simulink model "Rail_CtlLoop"  (R2016b)
settings: configuration reference "CodeGenConfigSet" (kept outside this file)
values from neighbouring files (symbols this model uses):
  FlSys_stDeflate_C = Calibration.Parameter    [init_Rail_CtlLoop.m]    (also in init_Rail_CtlLoop_SIL.m = Simulink.Parameter)
  Rail_dvolMeUnCtlInitI_CUR = Calibration.Parameter    [init_Rail_CtlLoop.m]    (also in init_Rail_CtlLoop_SIL.m = Simulink.Parameter)
  Rail_dvolMeUnCtlInitI_CURX = Calibration.Parameter    [init_Rail_CtlLoop.m]    (also in init_Rail_CtlLoop_SIL.m = Simulink.Parameter)
  Rail_dvolMeUnCtlLoLim_C = Calibration.Parameter    [init_Rail_CtlLoop.m]    (also in init_Rail_CtlLoop_SIL.m = Simulink.Parameter)
  Rail_dvolOff_C = Calibration.Parameter    [init_Rail_CtlLoop.m]    (also in init_Rail_CtlLoop_SIL.m = Simulink.Parameter)
  Rail_dvolPRVCtlOfs_C = Calibration.Parameter    [init_Rail_CtlLoop.m]    (also in init_Rail_CtlLoop_SIL.m = Simulink.Parameter)
  Rail_dvolStrt_MAP = Calibration.Parameter    [init_Rail_CtlLoop.m]    (also in init_Rail_CtlLoop_SIL.m = Simulink.Parameter)
  Rail_dvolStrt_MAPX = Calibration.Parameter    [init_Rail_CtlLoop.m]    (also in init_Rail_CtlLoop_SIL.m = Simulink.Parameter)
  Rail_dvolStrt_MAPY = Calibration.Parameter    [init_Rail_CtlLoop.m]    (also in init_Rail_CtlLoop_SIL.m = Simulink.Parameter)
  Rail_nCloseCtl_C = Calibration.Parameter    [init_Rail_CtlLoop.m]    (also in init_Rail_CtlLoop_SIL.m = Simulink.Parameter)
  Rail_nMeUnFrzI_C = Calibration.Parameter    [init_Rail_CtlLoop.m]    (also in init_Rail_CtlLoop_SIL.m = Simulink.Parameter)
  Rail_nOpnCtl_C = Calibration.Parameter    [init_Rail_CtlLoop.m]    (also in init_Rail_CtlLoop_SIL.m = Simulink.Parameter)
  Rail_nStrtLoPress_C = Calibration.Parameter    [init_Rail_CtlLoop.m]    (also in init_Rail_CtlLoop_SIL.m = Simulink.Parameter)
  Rail_numRevPlaus_C = Calibration.Parameter    [init_Rail_CtlLoop.m]    (also in init_Rail_CtlLoop_SIL.m = Simulink.Parameter)
  Rail_pCloseCtl_C = Calibration.Parameter    [init_Rail_CtlLoop.m]    (also in init_Rail_CtlLoop_SIL.m = Simulink.Parameter)
  Rail_pDiffCloseCtl_C = Calibration.Parameter    [init_Rail_CtlLoop.m]    (also in init_Rail_CtlLoop_SIL.m = Simulink.Parameter)
  Rail_pDvtFltMin_C = Calibration.Parameter    [init_Rail_CtlLoop.m]    (also in init_Rail_CtlLoop_SIL.m = Simulink.Parameter)
  Rail_pMeUnCtlIWinNeg_C = Calibration.Parameter    [init_Rail_CtlLoop.m]    (also in init_Rail_CtlLoop_SIL.m = Simulink.Parameter)
  Rail_pMeUnCtlIWinPos_C = Calibration.Parameter    [init_Rail_CtlLoop.m]    (also in init_Rail_CtlLoop_SIL.m = Simulink.Parameter)
  Rail_pMeUnCtlPWinNeg_C = Calibration.Parameter    [init_Rail_CtlLoop.m]    (also in init_Rail_CtlLoop_SIL.m = Simulink.Parameter)
  Rail_pMeUnCtlPWinPos_C = Calibration.Parameter    [init_Rail_CtlLoop.m]    (also in init_Rail_CtlLoop_SIL.m = Simulink.Parameter)
  Rail_pOpnCtl_C = Calibration.Parameter    [init_Rail_CtlLoop.m]    (also in init_Rail_CtlLoop_SIL.m = Simulink.Parameter)
  Rail_stCtlLoopSel_C = Calibration.Parameter    [init_Rail_CtlLoop.m]    (also in init_Rail_CtlLoop_SIL.m = Simulink.Parameter)
  Rail_swtPress_C = Calibration.Parameter    [init_Rail_CtlLoop.m]    (also in init_Rail_CtlLoop_SIL.m = Simulink.Parameter)
  Rail_tiFrzIDel_C = Calibration.Parameter    [init_Rail_CtlLoop.m]    (also in init_Rail_CtlLoop_SIL.m = Simulink.Parameter)
undefined symbols (not defined in the file or in its folder): Rail_CtlLoop_DT, RailCtl_State_conv
libraries: CXLib x7
settings Model: Creator=lenovo  LastModifiedBy=liutao
settings ConfigSetRef: SourceLocation=Base Workspace

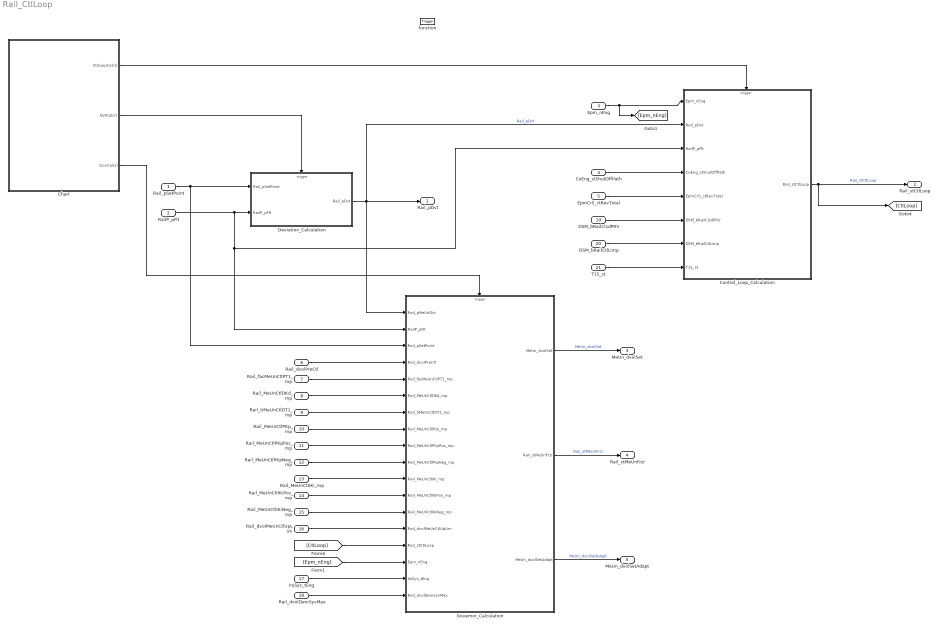
== system Rail_CtlLoop ==
  Rail_pSetPoint : Inport  Tag=bar  Description=Rail pressure setpoint  OutMin=-2500  OutMax=2500  OutDataTypeStr=RailPressure_bar
  RailP_pFlt : Inport  Tag=bar  Description=Maximum rail pressure of the last 10 sampling cycle  Port=2  OutMin=0  OutMax=2500  OutDataTypeStr=RailPressure_bar
  Epm_nEng : Inport  Tag=rpm  Description=Engine speed  Port=3  OutMin=0  OutMax=6000  OutDataTypeStr=EngSpeed_rpm
  CoEng_stShutOffPath : Inport  Description=Active shut-off paths resulting from active reversible,irreversible and afterrun shut-off paths  Port=4  OutMin=0  OutMax=65535  OutDataTypeStr=State_uint16
  EpmCrS_ctRevTotal : Inport  Description=Number of crankshaft rotations  Port=5  OutMin=0  OutMax=65535  OutDataTypeStr=Counter_num
  Rail_dvolPreCtl : Inport  Tag=mm^3/s  Description=Precontrol value for pressure governing by metering unit  Port=6  OutMin=-327680  OutMax=327670  OutDataTypeStr=FuelVol_mm3_s
  Rail_facMeUnCtlPT1_mp : Inport  Description=Time constant of the PT1 filter for pressure control by metering unit  Port=7  OutMin=0  OutMax=99.9985  OutDataTypeStr=PT_fac
  Rail_MeUnCtlDKd_mp : Inport  Description=D amplification for pressure control by metering unit  Port=8  OutMin=0  OutMax=15  OutDataTypeStr=Pid_Kp_Kd
  Rail_tiMeUnCtlDT1_mp : Inport  Tag=ms  Description=Time constant of the DT1 element for pressure control by metering unit  Port=9  OutMin=0  OutMax=65535  OutDataTypeStr=RailDT1_ms
  Rail_MeUnCtlPKp_mp : Inport  Description=P-Gain within the window  Port=10  OutMin=0  OutMax=15  OutDataTypeStr=Pid_Kp_Kd
  Rail_MeUnCtlPKpPos_mp : Inport  Description=P-gain above upper window border  Port=11  OutMin=0  OutMax=15  OutDataTypeStr=Pid_Kp_Kd
  Rail_MeUnCtlPKpNeg_mp : Inport  Description=P-gain below lower window border  Port=12  OutMin=0  OutMax=15  OutDataTypeStr=Pid_Kp_Kd
  Rail_MeUnCtlIKi_mp : Inport  Description=I-Gain within the window  Port=13  OutMin=0  OutMax=65  OutDataTypeStr=Pid_Ki
  Rail_MeUnCtlIKiPos_mp : Inport  Description=I-Gain above upper window border  Port=14  OutMin=0  OutMax=65  OutDataTypeStr=Pid_Ki
  Rail_MeUnCtlIKiNeg_mp : Inport  Description=I-Gain below upper window border  Port=15  OutMin=0  OutMax=65  OutDataTypeStr=Pid_Ki
  Rail_dvolMeUnCtlUpLim : Inport  Tag=mm^3/s  Description=Upper actuator value limit for pressure governing by metering unit  Port=16  OutMin=0  OutMax=327670  OutDataTypeStr=FuelVol_mm3_s
  InjSys_tEng : Inport  Tag=deg  Description=Engine temperature selected for the injection system  Port=17  OutMin=-1000  OutMax=1000  OutDataTypeStr=Temp_deg
  Rail_dvolDemSysMax : Inport  Tag=mm^3/s  Description=Volume flow requested overall for a maximum tolerated injection system  Port=18  OutMin=-327680  OutMax=327670  OutDataTypeStr=FuelVol_mm3_s
  DSM_bRailClsdPRV : Inport  Description=state of FId_RailClsdPRV  Port=19  OutMin=0  OutMax=1  OutDataTypeStr=boolean
  DSM_bRailCtlLimp : Inport  Description=state of FId_RailCtlLimp  Port=20  OutMin=0  OutMax=1  OutDataTypeStr=boolean
  T15_st : Inport  Description=Terminal 15 status after debouncing  Port=21  OutDataTypeStr=Enum: Switch_conv
  function : TriggerPort  TriggerType=function-call  VariantControl=Variant
  Chart : Stateflow chart
  Control_Loop_Calculation : Subsystem  TreatAsAtomicUnit=on
  Deviation_Calculation : Subsystem  TreatAsAtomicUnit=on
  Governor_Calculation : Subsystem  TreatAsAtomicUnit=on
  Rail_pDvt : Outport  Tag=bar  Description=Governor deviation of the rail pressure governor  OutMin=-2500  OutMax=2500  OutDataTypeStr=RailPressure_bar
  Rail_stCtlLoop : Outport  Description=State of the rail pressure governor control  Port=2  OutDataTypeStr=Enum: RailCtl_State_conv
  MeUn_dvolSet : Outport  Tag=mm^3/s  Description=Setpoint value (volume flow) of rail pressure governing  Port=3  OutMin=-327670  OutMax=327670  OutDataTypeStr=FuelVol_mm3_s
  Rail_stMeUnFrzI : Outport  Description=State bits for monitoring for a positive governor deviation  Port=4  OutMin=0  OutMax=1  OutDataTypeStr=Dsm
  MeUn_dvolSetAdapt : Outport  Tag=mm^3/s  Description=Correction value of the adaption of the metering unit  Port=5  OutMin=-327680  OutMax=327670  OutDataTypeStr=FuelVol_mm3_s
  wires:
  Deviation_Calculation/1(Rail_pDvt) -> Rail_pDvt/1, Control_Loop_Calculation/2(Rail_pDvt), Governor_Calculation/1(Rail_pMeUnDvt)  "Rail_pDvt"
  Governor_Calculation/1(MeUn_dvolSet) -> MeUn_dvolSet/1  "MeUn_dvolSet"
  Governor_Calculation/2(Rail_stMeUnFrzI) -> Rail_stMeUnFrzI/1  "Rail_stMeUnFrzI"
  DSM_bRailCtlLimp/1 -> Control_Loop_Calculation/7(DSM_bRailCtlLimp)
  DSM_bRailClsdPRV/1 -> Control_Loop_Calculation/6(DSM_bRailClsdPRV)
  EpmCrS_ctRevTotal/1 -> Control_Loop_Calculation/5(EpmCrS_ctRevTotal)
  [Epm_nEng] -> Governor_Calculation/16(Epm_nEng)
  Rail_dvolDemSysMax/1 -> Governor_Calculation/18(Rail_dvolDemSysMax)
  InjSys_tEng/1 -> Governor_Calculation/17(InjSys_tEng)
  [CtlLoop] -> Governor_Calculation/15(Rail_stCtlLoop)
  Rail_dvolMeUnCtlUpLim/1 -> Governor_Calculation/14(Rail_dvolMeUnCtlUpLim)
  Rail_MeUnCtlIKiNeg_mp/1 -> Governor_Calculation/13(Rail_MeUnCtlIKiNeg_mp)
  Rail_MeUnCtlIKiPos_mp/1 -> Governor_Calculation/12(Rail_MeUnCtlIKiPos_mp)
  Rail_MeUnCtlIKi_mp/1 -> Governor_Calculation/11(Rail_MeUnCtlIKi_mp)
  Rail_MeUnCtlPKpNeg_mp/1 -> Governor_Calculation/10(Rail_MeUnCtlPKpNeg_mp)
  Rail_MeUnCtlPKpPos_mp/1 -> Governor_Calculation/9(Rail_MeUnCtlPKpPos_mp)
  Rail_MeUnCtlPKp_mp/1 -> Governor_Calculation/8(Rail_MeUnCtlPKp_mp)
  Rail_tiMeUnCtlDT1_mp/1 -> Governor_Calculation/7(Rail_tiMeUnCtlDT1_mp)
  Rail_MeUnCtlDKd_mp/1 -> Governor_Calculation/6(Rail_MeUnCtlDKd_mp)
  Rail_facMeUnCtlPT1_mp/1 -> Governor_Calculation/5(Rail_facMeUnCtlPT1_mp)
  Rail_dvolPreCtl/1 -> Governor_Calculation/4(Rail_dvolPreCtl)
  Epm_nEng/1 -> [Epm_nEng], Control_Loop_Calculation/1(Epm_nEng)
  Chart/3(GovCalc()) -> Governor_Calculation/Trigger
  CoEng_stShutOffPath/1 -> Control_Loop_Calculation/4(CoEng_stShutOffPath)
  Rail_pSetPoint/1 -> Governor_Calculation/3(Rail_pSetPoint), Deviation_Calculation/1(Rail_pSetPoint)
  Chart/1(CtlLoopCalc()) -> Control_Loop_Calculation/Trigger
  Chart/2(DvtCalc()) -> Deviation_Calculation/Trigger
  RailP_pFlt/1 -> Governor_Calculation/2(RailP_pFlt), Control_Loop_Calculation/3(RailP_pFlt), Deviation_Calculation/2(RailP_pFlt)
  Governor_Calculation/3(MeUn_dvolSetAdapt) -> MeUn_dvolSetAdapt/1  "MeUn_dvolSetAdapt"
  Control_Loop_Calculation/1(Rail_stCtlLoop) -> Rail_stCtlLoop/1, [CtlLoop]  "Rail_stCtlLoop"
  T15_st/1 -> Control_Loop_Calculation/8(T15_st)

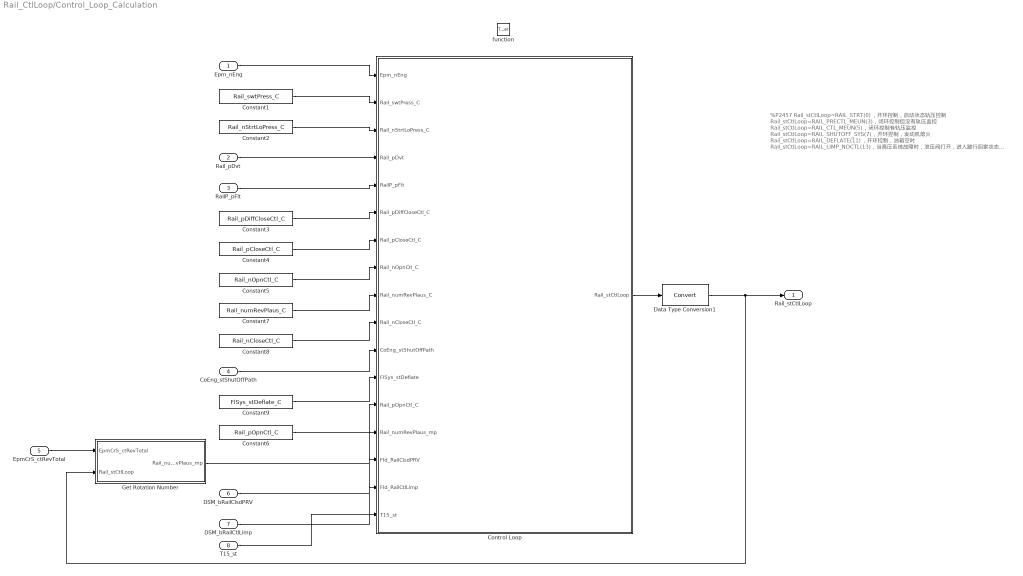
== system Rail_CtlLoop/Control_Loop_Calculation ==
  note: %P2457
      | Rail_stCtlLoop=RAIL_STRT(0)，开环控制，启动状态轨压控制
      | Rail_stCtlLoop=RAIL_PRECTL_MEUN(3)，闭环控制但没有轨压监控
      | Rail_stCtlLoop=RAIL_CTL_MEUN(5)，闭环控制有轨压监控
      | Rail_stCtlLoop=RAIL_SHUTOFF_SYS(7)，开环控制，发动机熄火
      | Rail_stCtlLoop=RAIL_DEFLATE(11)，开环控制，油箱空时
      | Rail_stCtlLoop=RAIL_LIMP_NOCTL(13)，当高压系统故障时，泄压阀打开，进入跛行回家状态
      | Rail_stCtlLoop=RAIL_LIMP_OPENCTL(14)，跛行回家没有故障时，进入开环控制，防止油温过高
      | %
  Epm_nEng : Inport
  Rail_pDvt : Inport  Port=2
  RailP_pFlt : Inport  Port=3
  CoEng_stShutOffPath : Inport  Port=4
  EpmCrS_ctRevTotal : Inport  Port=5
  DSM_bRailClsdPRV : Inport  Port=6
  DSM_bRailCtlLimp : Inport  Port=7
  T15_st : Inport  Port=8
  function : TriggerPort  TriggerType=function-call  VariantControl=Variant
  Constant1 : Constant  Value=Rail_swtPress_C  SampleTime=-1
  Constant2 : Constant  Value=Rail_nStrtLoPress_C  SampleTime=-1
  Constant3 : Constant  Value=Rail_pDiffCloseCtl_C  SampleTime=-1
  Constant4 : Constant  Value=Rail_pCloseCtl_C  SampleTime=-1
  Constant5 : Constant  Value=Rail_nOpnCtl_C  SampleTime=-1
  Constant6 : Constant  Value=Rail_pOpnCtl_C  SampleTime=-1
  Constant7 : Constant  Value=Rail_numRevPlaus_C  SampleTime=-1
  Constant8 : Constant  Value=Rail_nCloseCtl_C  SampleTime=-1
  Constant9 : Constant  Value=FlSys_stDeflate_C  SampleTime=-1
  Control Loop : Stateflow chart  TreatAsAtomicUnit=on
  Data Type Conversion1 : DataTypeConversion
  Get Rotation Number : Subsystem
  Rail_stCtlLoop : Outport
  wires:
  DSM_bRailCtlLimp/1 -> Control Loop/16(FId_RailCtlLimp)
  DSM_bRailClsdPRV/1 -> Control Loop/15(FId_RailClsdPRV)
  Get Rotation Number/1(Rail_numRevPlaus_mp) -> Control Loop/14(Rail_numRevPlaus_mp)
  CoEng_stShutOffPath/1 -> Control Loop/11(CoEng_stShutOffPath)
  Control Loop/1(Rail_stCtlLoop) -> Data Type Conversion1/1
  Constant6/1 -> Control Loop/13(Rail_pOpnCtl_C)
  Constant8/1 -> Control Loop/10(Rail_nCloseCtl_C)
  Constant7/1 -> Control Loop/9(Rail_numRevPlaus_C)
  Constant5/1 -> Control Loop/8(Rail_nOpnCtl_C)
  Constant4/1 -> Control Loop/7(Rail_pCloseCtl_C)
  Constant3/1 -> Control Loop/6(Rail_pDiffCloseCtl_C)
  Constant1/1 -> Control Loop/2(Rail_swtPress_C)
  Constant2/1 -> Control Loop/3(Rail_nStrtLoPress_C)
  Constant9/1 -> Control Loop/12(FlSys_stDeflate)
  RailP_pFlt/1 -> Control Loop/5(RailP_pFlt)
  Rail_pDvt/1 -> Control Loop/4(Rail_pDvt)
  Epm_nEng/1 -> Control Loop/1(Epm_nEng)
  EpmCrS_ctRevTotal/1 -> Get Rotation Number/1(EpmCrS_ctRevTotal)
  Data Type Conversion1/1 -> Get Rotation Number/2(Rail_stCtlLoop), Rail_stCtlLoop/1
  T15_st/1 -> Control Loop/17(T15_st)

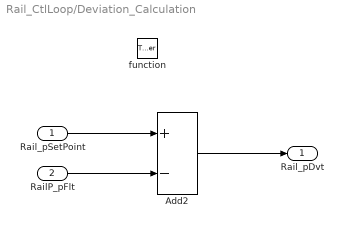
== system Rail_CtlLoop/Deviation_Calculation ==
  Rail_pSetPoint : Inport
  RailP_pFlt : Inport  Port=2
  function : TriggerPort  TriggerType=function-call  VariantControl=Variant
  Add2 : Sum  Inputs=+-  InputSameDT=on
  Rail_pDvt : Outport
  wires:
  Add2/1 -> Rail_pDvt/1
  RailP_pFlt/1 -> Add2/2
  Rail_pSetPoint/1 -> Add2/1

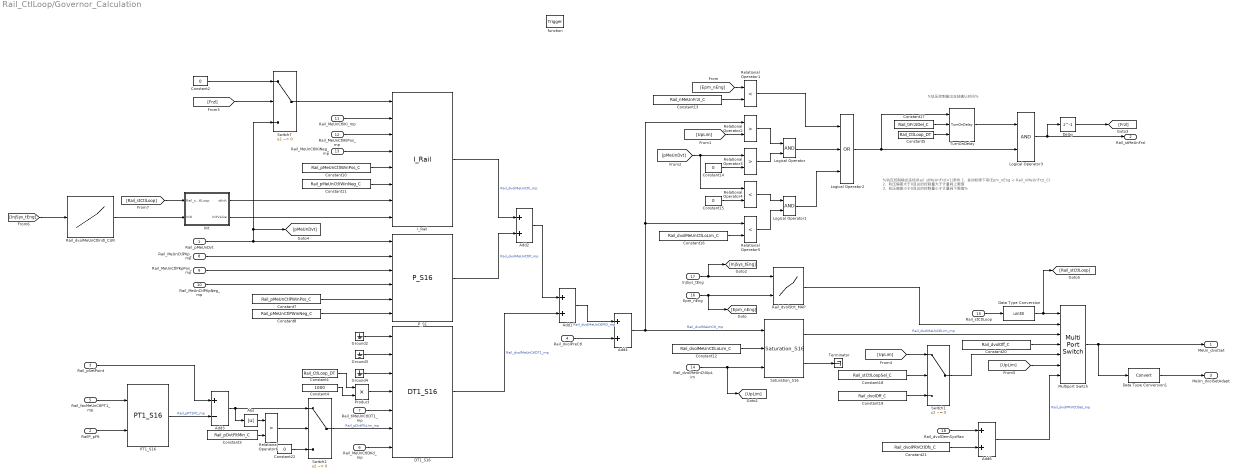
== system Rail_CtlLoop/Governor_Calculation ==
  note: %轨压控制输出冻结(Rail_stMeUnFrzI=1)条件
      | 1、发动机停下来(Epm_nEng < Rail_nMeUnFrzI_C)
      | 2、轨压偏差大于0且总的控制量大于计量阀上限值
      | 3、轨压偏差小于0且总的控制量小于计量阀下限值%
  note: %轨压控制输出冻结确认时间%
  Rail_pMeUnDvt : Inport
  RailP_pFlt : Inport  Port=2
  Rail_pSetPoint : Inport  Port=3
  Rail_dvolPreCtl : Inport  Port=4
  Rail_facMeUnCtlPT1_mp : Inport  Port=5
  Rail_MeUnCtlDKd_mp : Inport  Port=6
  Rail_tiMeUnCtlDT1_mp : Inport  Port=7
  Rail_MeUnCtlPKp_mp : Inport  Port=8
  Rail_MeUnCtlPKpPos_mp : Inport  Port=9
  Rail_MeUnCtlPKpNeg_mp : Inport  Port=10
  Rail_MeUnCtlIKi_mp : Inport  Port=11
  Rail_MeUnCtlIKiPos_mp : Inport  Port=12
  Rail_MeUnCtlIKiNeg_mp : Inport  Port=13
  Rail_dvolMeUnCtlUpLim : Inport  Port=14
  Rail_stCtlLoop : Inport  Port=15
  Epm_nEng : Inport  Port=16
  InjSys_tEng : Inport  Port=17
  Rail_dvolDemSysMax : Inport  Port=18
  function : TriggerPort  TriggerType=function-call  VariantControl=Variant
  Abs : Abs
  Add1 : Sum  SaturateOnIntegerOverflow=on  InputSameDT=on
  Add2 : Sum  SaturateOnIntegerOverflow=on  InputSameDT=on
  Add3 : Sum  Inputs=+-  InputSameDT=on
  Add4 : Sum  InputSameDT=on
  Add6 : Sum  InputSameDT=on
  Constant1 : Constant  Value=Rail_CtlLoop_DT  OutDataTypeStr=uint32
  Constant10 : Constant  Value=Rail_pMeUnCtlIWinPos_C  SampleTime=-1
  Constant11 : Constant  Value=Rail_pMeUnCtlIWinNeg_C  SampleTime=-1
  Constant12 : Constant  Value=Rail_dvolMeUnCtlLoLim_C  SampleTime=-1
  Constant13 : Constant  Value=Rail_nMeUnFrzI_C  SampleTime=-1
  Constant{2,14..15,22} (4 alike) : Constant  Value=0  OutDataTypeStr=Inherit: Inherit via back propagation  SampleTime=-1
  Constant16 : Constant  Value=Rail_dvolMeUnCtlLoLim_C  SampleTime=-1  LockScale=on
  Constant17 : Constant  Value=Rail_tiFrzIDel_C
  Constant18 : Constant  Value=Rail_stCtlLoopSel_C  SampleTime=-1
  Constant19 : Constant  Value=Rail_dvolOff_C  SampleTime=-1
  Constant20 : Constant  Value=Rail_dvolOff_C  SampleTime=-1
  Constant21 : Constant  Value=Rail_dvolPRVCtlOfs_C  SampleTime=-1
  Constant3 : Constant  Value=Rail_pDvtFltMin_C  SampleTime=-1
  Constant4 : Constant  Value=1000  OutDataTypeStr=uint16
  Constant5 : Constant  Value=Rail_CtlLoop_DT  OutDataTypeStr=uint32
  Constant7 : Constant  Value=Rail_pMeUnCtlPWinPos_C  SampleTime=-1
  Constant8 : Constant  Value=Rail_pMeUnCtlPWinNeg_C  SampleTime=-1
  DT1_S16 : CXLib/DT1_S16
  Data Type Conversion : DataTypeConversion  OutDataTypeStr=uint8
  Data Type Conversion1 : DataTypeConversion
  Delay : Delay  DelayLength=1  InitialCondition=0
  Ground2 : Ground
  Ground3 : Ground
  Ground4 : Ground
  I_Rail : CXLib/I_Rail
  Init : Subsystem
  Logical Operator : Logic  AllPortsSameDT=off  OutDataTypeStr=boolean
  Logical Operator1 : Logic  AllPortsSameDT=off  OutDataTypeStr=boolean
  Logical Operator2 : Logic  Operator=OR  Inputs=3  AllPortsSameDT=off  OutDataTypeStr=boolean
  Logical Operator3 : Logic  AllPortsSameDT=off  OutDataTypeStr=boolean
  Multiport Switch : MultiPortSwitch  DataPortOrder=Specify indices  DataPortIndices={0,[3,5],7,11,13,14}  DiagnosticForDefault=None  InputSameDT=on
  PT1_S16 : CXLib/PT1_S16
  P_S1 : CXLib/P_S16
  Product : Product  OutDataTypeStr=uint32
  Rail_dvolMeUnCtlInitI_CUR : Lookup_n-D  NumberOfTableDimensions=1  BreakpointsForDimension1=Rail_dvolMeUnCtlInitI_CURX  IndexSearchMethod=Linear search  BeginIndexSearchUsingPreviousIndexResult=on  Table=Rail_dvolMeUnCtlInitI_CUR  ExtrapMethod=Clip  UseLastTableValue=on  InternalRulePriority=Speed  OutDataTypeStr=Inherit: Inherit via back propagation  SaturateOnIntegerOverflow=on
  Rail_dvolStrt_MAP : Lookup_n-D  BreakpointsForDimension1=Rail_dvolStrt_MAPY  BreakpointsForDimension2=Rail_dvolStrt_MAPX  IndexSearchMethod=Linear search  BeginIndexSearchUsingPreviousIndexResult=on  Table=Rail_dvolStrt_MAP  ExtrapMethod=Clip  UseLastTableValue=on  InternalRulePriority=Speed  OutDataTypeStr=Inherit: Inherit via back propagation  RndMeth=Simplest  SaturateOnIntegerOverflow=on
  Relational Operator1 : RelationalOperator  Operator=<  OutDataTypeStr=boolean  RndMeth=Nearest  InputSameDT=on
  Relational Operator2 : RelationalOperator  Operator=>  OutDataTypeStr=boolean  RndMeth=Nearest  InputSameDT=on
  Relational Operator3 : RelationalOperator  Operator=>  OutDataTypeStr=boolean  RndMeth=Nearest  InputSameDT=on
  Relational Operator4 : RelationalOperator  Operator=<  OutDataTypeStr=boolean  RndMeth=Nearest  InputSameDT=on
  Relational Operator5 : RelationalOperator  Operator=<  OutDataTypeStr=boolean  RndMeth=Nearest  InputSameDT=on
  Relational Operator6 : RelationalOperator  Operator=>  OutDataTypeStr=boolean  RndMeth=Nearest  InputSameDT=on
  Saturation_S16 : CXLib/Saturation_S16
  Switch1 : Switch  Criteria=u2 ~= 0  InputSameDT=on
  Switch2 : Switch  Criteria=u2 ~= 0  InputSameDT=on
  Switch7 : Switch  Criteria=u2 ~= 0  InputSameDT=on
  Terminator : Terminator
  TurnOnDelay : CXLib/TurnOnDelay
  MeUn_dvolSet : Outport
  Rail_stMeUnFrzI : Outport  Port=2
  MeUn_dvolSetAdapt : Outport  Tag=mm^3/s  Description=Correction value of the adaption of the metering unit  Port=3
  wires:
  Constant5/1 -> TurnOnDelay/3
  DT1_S16/1 -> Add1/2  "Rail_dvolMeUnCtlDT1_mp"
  Constant12/1 -> Saturation_S16/2
  Rail_dvolStrt_MAP/1 -> Multiport Switch/2
  Switch7/1 -> I_Rail/1
  Abs/1 -> Relational Operator6/1
  Add3/1 -> Switch2/1, Abs/1
  Switch1/1 -> Multiport Switch/5
  [UpLim] -> Multiport Switch/6
  Constant20/1 -> Multiport Switch/4
  Constant22/1 -> Switch2/3
  Relational Operator6/1 -> Switch2/2
  Switch2/1 -> DT1_S16/6  "Rail_pDvtFltLim_mp"
  Delay/1 -> [Frzl]
  Add6/1 -> Multiport Switch/7  "Rail_dvolPRVCtlSet_mp"
  Constant21/1 -> Add6/2
  Rail_dvolDemSysMax/1 -> Add6/1
  Constant19/1 -> Switch1/3
  [UpLim] -> Switch1/1
  Constant18/1 -> Switch1/2
  [Frzl] -> Switch7/2
  Logical Operator3/1 -> Rail_stMeUnFrzI/1, Delay/1
  Constant17/1 -> TurnOnDelay/2
  TurnOnDelay/1 -> Logical Operator3/1
  Logical Operator2/1 -> Logical Operator3/2, TurnOnDelay/1
  Logical Operator1/1 -> Logical Operator2/3
  Logical Operator/1 -> Logical Operator2/2
  Relational Operator1/1 -> Logical Operator2/1
  Relational Operator5/1 -> Logical Operator1/2
  Relational Operator4/1 -> Logical Operator1/1
  Constant16/1 -> Relational Operator5/2
  Constant15/1 -> Relational Operator4/2
  Relational Operator3/1 -> Logical Operator/2
  Relational Operator2/1 -> Logical Operator/1
  [pMeUnDvt] -> Relational Operator3/1, Relational Operator4/1
  Constant14/1 -> Relational Operator3/2
  [UpLim] -> Relational Operator2/2
  Constant13/1 -> Relational Operator1/2
  [Epm_nEng] -> Relational Operator1/1
  Multiport Switch/1 -> Data Type Conversion1/1, MeUn_dvolSet/1
  InjSys_tEng/1 -> Rail_dvolStrt_MAP/1, [InjSys_tEng]
  Epm_nEng/1 -> Rail_dvolStrt_MAP/2, [Epm_nEng]
  Rail_stCtlLoop/1 -> Data Type Conversion/1
  Saturation_S16/1 -> Multiport Switch/3  "Rail_dvolMeUnCtlLim_mp"
  Saturation_S16/2 -> Terminator/1
  Rail_dvolMeUnCtlUpLim/1 -> [UpLim], Saturation_S16/3
  Init/2(InitValue) -> I_Rail/8
  Init/1(stInit) -> I_Rail/7
  Constant11/1 -> I_Rail/6
  Constant10/1 -> I_Rail/5
  Rail_MeUnCtlIKiNeg_mp/1 -> I_Rail/4
  Rail_MeUnCtlIKiPos_mp/1 -> I_Rail/3
  Rail_MeUnCtlIKi_mp/1 -> I_Rail/2
  Constant8/1 -> P_S1/6
  Constant7/1 -> P_S1/5
  Rail_MeUnCtlPKp_mp/1 -> P_S1/2
  Rail_MeUnCtlPKpPos_mp/1 -> P_S1/3
  Rail_MeUnCtlPKpNeg_mp/1 -> P_S1/4
  Ground3/1 -> DT1_S16/2
  Ground4/1 -> DT1_S16/3
  Ground2/1 -> DT1_S16/1
  Rail_tiMeUnCtlDT1_mp/1 -> DT1_S16/5
  Rail_MeUnCtlDKd_mp/1 -> DT1_S16/7
  Product/1 -> DT1_S16/4
  Constant3/1 -> Relational Operator6/2
  Rail_facMeUnCtlPT1_mp/1 -> PT1_S16/1
  Add4/1 -> Saturation_S16/1, Relational Operator5/1, Relational Operator2/1  "Rail_dvolMeUnCtl_mp"
  Rail_dvolPreCtl/1 -> Add4/2
  Add1/1 -> Add4/1  "Rail_dvolMeUnCtlPID_mp"
  RailP_pFlt/1 -> PT1_S16/2
  PT1_S16/1 -> Add3/2  "Rail_pPT1Flt_mp"
  Rail_pSetPoint/1 -> Add3/1
  Add2/1 -> Add1/1
  P_S1/1 -> Add2/2  "Rail_dvolMeUnCtlP_mp"
  I_Rail/1 -> Add2/1  "Rail_dvolMeUnCtlI_mp"
  Constant2/1 -> Switch7/1
  Rail_pMeUnDvt/1 -> [pMeUnDvt], Switch7/3, P_S1/1
  Data Type Conversion/1 -> Multiport Switch/1, [Rail_stCtlLoop]
  [Rail_stCtlLoop] -> Init/1(Rail_stCtlLoop)
  [InjSys_tEng] -> Rail_dvolMeUnCtlInitI_CUR/1
  Rail_dvolMeUnCtlInitI_CUR/1 -> Init/2(InitI)
  Data Type Conversion1/1 -> MeUn_dvolSetAdapt/1
  Constant1/1 -> Product/1
  Constant4/1 -> Product/2

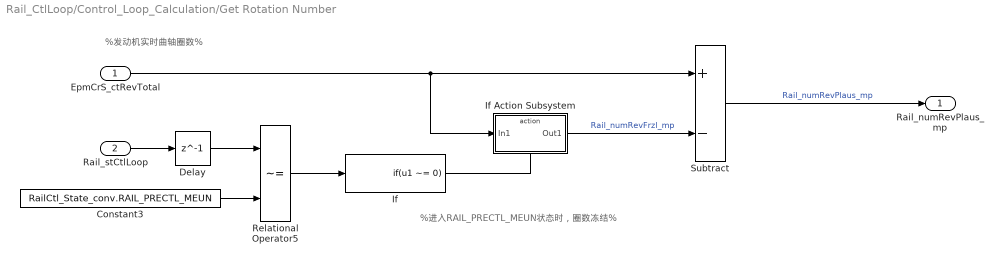
== system Rail_CtlLoop/Control_Loop_Calculation/Get Rotation Number ==
  note: %进入RAIL_PRECTL_MEUN状态时，圈数冻结%
  note: %发动机实时曲轴圈数%
  EpmCrS_ctRevTotal : Inport
  Rail_stCtlLoop : Inport  Port=2
  Constant3 : Constant  Value=RailCtl_State_conv.RAIL_PRECTL_MEUN  SampleTime=-1
  Delay : Delay  DelayLength=1  InitialCondition=RailCtl_State_conv.RAIL_STRT
  If : If  IfExpression=u1 ~= 0  ShowElse=off
  If Action Subsystem : Subsystem  TreatAsAtomicUnit=on
  Relational Operator5 : RelationalOperator  Operator=~=  OutDataTypeStr=boolean  RndMeth=Round  InputSameDT=on
  Subtract : Sum  Inputs=+-  OutDataTypeStr=Inherit: Inherit via back propagation  SaturateOnIntegerOverflow=on  InputSameDT=on
  Rail_numRevPlaus_mp : Outport
  wires:
  Delay/1 -> Relational Operator5/1
  Rail_stCtlLoop/1 -> Delay/1
  Constant3/1 -> Relational Operator5/2
  EpmCrS_ctRevTotal/1 -> Subtract/1, If Action Subsystem/1(In1)
  If/1 -> If Action Subsystem/Action
  If Action Subsystem/1(Out1) -> Subtract/2  "Rail_numRevFrzl_mp"
  Relational Operator5/1 -> If/1
  Subtract/1 -> Rail_numRevPlaus_mp/1  "Rail_numRevPlaus_mp"

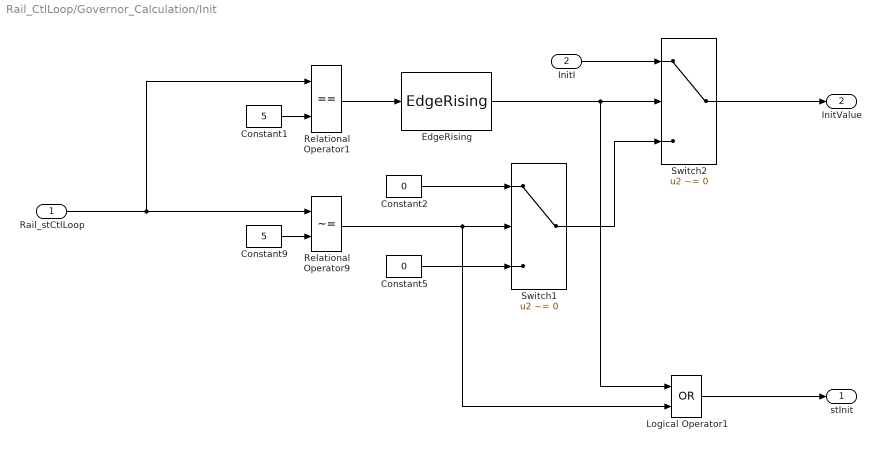
== system Rail_CtlLoop/Governor_Calculation/Init ==
  Rail_stCtlLoop : Inport
  InitI : Inport  Port=2
  Constant1 : Constant  Value=5  OutDataTypeStr=uint8  SampleTime=-1
  Constant2 : Constant  Value=0  OutDataTypeStr=FuelVol_mm3_s  SampleTime=-1
  Constant5 : Constant  Value=0  OutDataTypeStr=FuelVol_mm3_s  SampleTime=-1
  Constant9 : Constant  Value=5  OutDataTypeStr=uint8  SampleTime=-1
  EdgeRising : CXLib/EdgeRising
  Logical Operator1 : Logic  Operator=OR  AllPortsSameDT=off  OutDataTypeStr=boolean
  Relational Operator1 : RelationalOperator  Operator===  OutDataTypeStr=boolean  RndMeth=Nearest
  Relational Operator9 : RelationalOperator  Operator=~=  OutDataTypeStr=boolean  RndMeth=Nearest
  Switch1 : Switch  Criteria=u2 ~= 0  InputSameDT=on
  Switch2 : Switch  Criteria=u2 ~= 0  InputSameDT=on
  stInit : Outport
  InitValue : Outport  Port=2
  wires:
  Constant5/1 -> Switch1/3
  Switch2/1 -> InitValue/1
  Logical Operator1/1 -> stInit/1
  Switch1/1 -> Switch2/3
  InitI/1 -> Switch2/1
  EdgeRising/1 -> Switch2/2, Logical Operator1/1
  Relational Operator1/1 -> EdgeRising/1
  Constant2/1 -> Switch1/1
  Constant1/1 -> Relational Operator1/2
  Rail_stCtlLoop/1 -> Relational Operator9/1, Relational Operator1/1
  Constant9/1 -> Relational Operator9/2
  Relational Operator9/1 -> Switch1/2, Logical Operator1/2

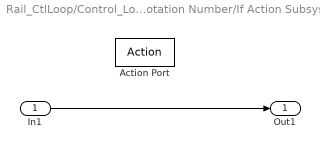
== system Rail_CtlLoop/Control_Loop_Calculation/Get Rotation Number/If Action Subsystem ==
  In1 : Inport
  Action Port : ActionPort  ActionType=then
  Out1 : Outport
  wires:
  In1/1 -> Out1/1

== stateflow chart Rail_CtlLoop/Control_Loop_Calculation/Control Loop ==
  state RAIL_SHUTOFF_SYS
    during:Rail_stCtlLoop = uint8(7);
  state WORKING
    state RAIL_LIMP_OPENCTL
      during:Rail_stCtlLoop = uint8(14);
    state RAIL_STRT
      during:Rail_stCtlLoop = uint8(0);
    state RAIL_PRECTL_MEUN
      during:Rail_stCtlLoop = uint8(3);
    state RAIL_LIMP_NOCTL
      during:Rail_stCtlLoop = uint8(13);
    state RAIL_CTL_MEUN
      during:Rail_stCtlLoop = uint8(5);
    state RAIL_DEFLATE
      during:Rail_stCtlLoop = uint8(11);
    RAIL_LIMP_NOCTL -> RAIL_LIMP_OPENCTL : [FId_RailCtlLimp > 0]
    RAIL_LIMP_OPENCTL -> RAIL_PRECTL_MEUN [order 2] : [(FId_RailCtlLimp > 0)&&...
        | (FId_RailClsdPRV > 0)]
    RAIL_LIMP_OPENCTL -> RAIL_LIMP_NOCTL [order 1] : [FId_RailCtlLimp == 0]
    RAIL_PRECTL_MEUN -> RAIL_STRT [order 1] : [(Epm_nEng <= Rail_nOpnCtl_C)&&...
        | (RailP_pFlt < Rail_pOpnCtl_C)]
    RAIL_STRT -> RAIL_PRECTL_MEUN [order 1] : [(Epm_nEng > Rail_nStrtLoPress_C)||...
        | ((Rail_swtPress_C == 1)&&(Rail_pDvt < Rail_pDiffCloseCtl_C))||...
        | ((Rail_swtPress_C == 0)&&(RailP_pFlt >= Rail_pCloseCtl_C))]
    RAIL_PRECTL_MEUN -> RAIL_LIMP_NOCTL [order 3] : [FId_RailClsdPRV == 0]
    RAIL_DEFLATE -> RAIL_STRT [order 1] : [(FlSys_stDeflate & uint8(2)) >0]
    RAIL_STRT -> RAIL_DEFLATE [order 2] : [((FlSys_stDeflate & uint8(1))==1)&&...
        | ((FlSys_stDeflate & uint8(2))==0)]
    RAIL_CTL_MEUN -> RAIL_STRT [order 1] : [(Epm_nEng <= Rail_nOpnCtl_C)&&...
        | (RailP_pFlt < Rail_pOpnCtl_C)]
    RAIL_PRECTL_MEUN -> RAIL_CTL_MEUN [order 2] : [Rail_numRevPlaus_mp >= Rail_numRevPlaus_C]
    RAIL_DEFLATE -> RAIL_LIMP_NOCTL [order 2] : [FId_RailClsdPRV == 0]
    RAIL_CTL_MEUN -> RAIL_LIMP_NOCTL [order 2] : [FId_RailClsdPRV == 0]
  WORKING -> RAIL_SHUTOFF_SYS : [(((CoEng_stShutOffPath & uint8(4)) > 0)&&...
      | (Rail_stCtlLoop ~= 7))||T15_st==Switch_conv.OFF]
  RAIL_SHUTOFF_SYS -> RAIL_STRT [order 2] : [((CoEng_stShutOffPath&uint8(4)) == 0)&&...
      | (Epm_nEng <= Rail_nCloseCtl_C)&&T15_st==Switch_conv.ON]
  RAIL_SHUTOFF_SYS -> RAIL_PRECTL_MEUN [order 1] : [((CoEng_stShutOffPath&uint8(4)) == 0)&&...
      | (Epm_nEng > Rail_nCloseCtl_C)&&T15_st==Switch_conv.ON ]
  (default) -> RAIL_STRT
  data: Rail_stCtlLoop output uint8; Epm_nEng input; Rail_swtPress_C input boolean; Rail_nStrtLoPress_C input; Rail_pDvt input; RailP_pFlt input; Rail_pDiffCloseCtl_C input; Rail_pCloseCtl_C input; Rail_nOpnCtl_C input; Rail_numRevPlaus_C input; Rail_nCloseCtl_C input; CoEng_stShutOffPath input; FlSys_stDeflate input uint8; Rail_pOpnCtl_C input; Rail_numRevPlaus_mp input; FId_RailClsdPRV input; FId_RailCtlLimp input; T15_st input

== stateflow chart Rail_CtlLoop/Chart ==
  (default) -> (junction 2)
  (junction 2) -> (junction 4) : {DvtCalc;}
  (junction 4) -> (junction 6) : {CtlLoopCalc;}
  (junction 6) -> (junction 9) : {GovCalc;}
  events: CtlLoopCalc output FUNCTION_CALL_EVENT; DvtCalc output FUNCTION_CALL_EVENT; GovCalc output FUNCTION_CALL_EVENT
